simulink model "Zero"  (R2021b)
settings: Solver=VariableStepAuto  StartTime=0.0  StopTime=10.0  RelTol=1e-3
undefined symbols (not defined in the file): Newton, Raphson
libraries: simulink x12, slpidlib x1
settings Model: SimulationMode=accelerator  Creator=user  LastModifiedBy=cemery

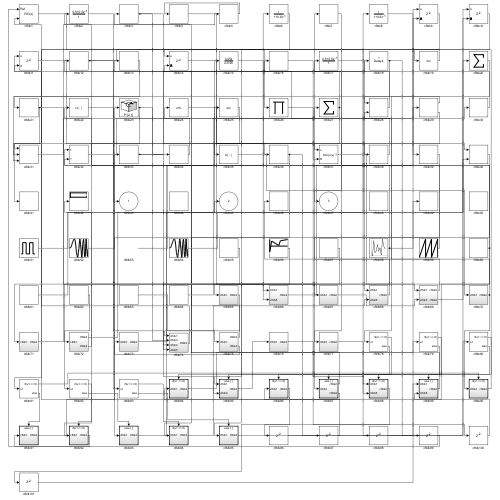
[thumbnail: Simulink's stored preview of the top-level diagram]
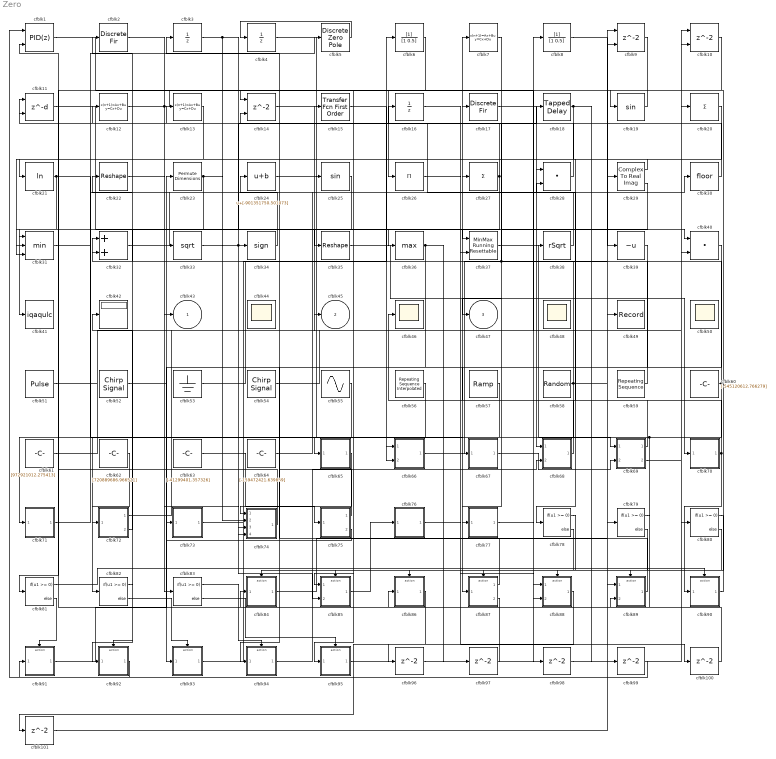
== system Zero ==
  cfblk1 : slpidlib/PID Controller (2DOF)  Controller=PID  Form=Parallel  TimeDomain=Discrete-time  UseExternalTs=off  SampleTime=1  IntegratorMethod=Forward Euler  FilterMethod=Forward Euler  ControllerParametersSource=internal  P=1  I=1  D=0  UseFilter=on  N=100  b=1  c=1  TunerSelectOption=Transfer Function Based (PID Tuner App)  InitialConditionSource=internal  InitialConditionForIntegrator=0  InitialConditionForFilter=0  DifferentiatorICPrevScaledInput=0  ExternalReset=none  TrackingMode=off  Kt=1  LimitOutput=off  SatLimitsSource=internal  UpperSaturationLimit=inf  LowerSaturationLimit=-inf  LinearizeAsGain=off  AntiWindupMode=none  Kb=1  POutMin=[]  POutMax=[]  IOutMin=[]  IOutMax=[]  DOutMin=[]  DOutMax=[]  NOutMin=[]  NOutMax=[]  bOutMin=[]  bOutMax=[]  cOutMin=[]  cOutMax=[]  SumOutMin=[]  SumOutMax=[]  SaturationOutMin=[]  SaturationOutMax=[]  PParamMin=[]  PParamMax=[]  IParamMin=[]  IParamMax=[]  DParamMin=[]  DParamMax=[]  NParamMin=[]  NParamMax=[]  bParamMin=[]  bParamMax=[]  cParamMin=[]  cParamMax=[]  KbParamMin=[]  KbParamMax=[]  KtParamMin=[]  KtParamMax=[]  KbOutMin=[]  KbOutMax=[]  KtOutMin=[]  KtOutMax=[]  IntegratorOutMin=[]  IntegratorOutMax=[]  FilterOutMin=[]  FilterOutMax=[]  SumI1OutMin=[]  SumI1OutMax=[]  SumI2OutMin=[]  SumI2OutMax=[]  SumI3OutMin=[]  SumI3OutMax=[]  SumI4OutMin=[]  SumI4OutMax=[]  SumDOutMin=[]  SumDOutMax=[]  Sum1OutMin=[]  Sum1OutMax=[]  Sum2OutMin=[]  Sum2OutMax=[]  Sum3OutMin=[]  Sum3OutMax=[]  DifferentiatorOutMin=[]  DifferentiatorOutMax=[]  FilterDiffOutCoefMin=[]  FilterDiffOutCoefMax=[]  ReciprocalOutMin=[]  ReciprocalOutMax=[]  SumDenOutMin=[]  SumDenOutMax=[]  SumNumOutMin=[]  SumNumOutMax=[]  DivideOutMin=[]  DivideOutMax=[]  UdiffTsProdOutMin=[]  UdiffTsProdOutMax=[]  NTsProdOutMin=[]  NTsProdOutMax=[]  UintegralTsProdOutMin=[]  UintegralTsProdOutMax=[]  UngainTsProdOutMin=[]  UngainTsProdOutMax=[]  IntegratorContinuousStateAttributes=''  IntegratorStateMustResolveToSignalObject=off  IntegratorRTWStateStorageClass=Auto  FilterContinuousStateAttributes=''  FilterStateMustResolveToSignalObject=off  FilterRTWStateStorageClass=Auto  ParallelPVariant=InternalParameters  IdealPVariant=Disabled  IVariant=InternalParameters  DVariant=InternalParameters  bVariant=InternalParameters  cVariant=InternalParameters  IntegratorVariant=Discrete  SatVariant=Disabled  AWVariant=Passthrough  PCopyVariant=Disabled  TRVariant=Disabled  FdbkBlocksVariant=Forward  IdealPFdbkVariant=Disabled  SatFdbkVariant=Disabled  DerivativeFilterVariant=ForwardEulerFilter  NVariant=InternalParameters  NCopyVariant=Disabled  FilterICVariant=InternalICsFilter  IntegratorICVariant=InternalICs  ExternalResetVariant=Disabled  TRSumVariant=Passthrough  SumFdbkVariant=Disabled  SumVariant=Sum_PID  TsampFilterVariant=InternalTs  TsampNgainVariant=Passthrough  TsampIntegralVariant=Passthrough  ExternalSaturationOutDataTypeStr=Inherit: Same as second input
      settings: SourceProductBaseCode=SL
  cfblk10 : Delay  ShowEnablePort=on  SampleTime=1
      settings: InputPortMap=u0,e6
  cfblk{96..101} (6 alike) : Delay  SampleTime=1
  cfblk11 : Delay  DelayLengthSource=Input port  SampleTime=1
      settings: InputPortMap=u0,p1
  cfblk12 : DiscreteStateSpace
  cfblk13 : DiscreteStateSpace
  cfblk14 : Delay  ShowEnablePort=on  SampleTime=1
      settings: InputPortMap=u0,e6
  cfblk15 : simulink/Discrete/Transfer Fcn First Order  PoleZ=0.95  ICPrevOutput=0.0  DoSatur=off
  cfblk16 : UnitDelay  HasFrameUpgradeWarning=on
  cfblk17 : DiscreteFir  SampleTime=1
  cfblk18 : simulink/Discrete/Tapped Delay  vinit=0.0  samptime=-1  NumDelays=1  DelayOrder=Oldest  includeCurrent=off
  cfblk19 : Trigonometry
  cfblk2 : DiscreteFir  SampleTime=1
  cfblk20 : Sum  Inputs=+
  cfblk21 : Math  Operator=log  SaturateOnIntegerOverflow=on
  cfblk22 : Reshape
  cfblk23 : PermuteDimensions
  cfblk24 : Bias  Bias=[-901351750.501073]
  cfblk25 : Trigonometry
  cfblk26 : Product  Inputs=*
  cfblk27 : Sum  Inputs=+
  cfblk28 : DotProduct  InputSameDT=on  OutDataTypeStr=Inherit: Inherit via internal rule
  cfblk29 : ComplexToRealImag
  cfblk3 : UnitDelay  HasFrameUpgradeWarning=on
  cfblk30 : Rounding
  cfblk31 : MinMax  Inputs=3
  cfblk32 : Sum
  cfblk33 : Sqrt  SaturateOnIntegerOverflow=on
  cfblk34 : Signum
  cfblk35 : Reshape
  cfblk36 : MinMax  Function=max
  cfblk37 : simulink/Math Operations/MinMax Running Resettable  Function=min  vinit=0.0
  cfblk38 : Sqrt  Operator=rSqrt  AlgorithmType=Newton-Raphson  SaturateOnIntegerOverflow=on
  cfblk39 : UnaryMinus
  cfblk4 : UnitDelay  HasFrameUpgradeWarning=on
  cfblk40 : DotProduct  InputSameDT=on  OutDataTypeStr=Inherit: Inherit via internal rule
  cfblk41 : ToWorkspace  VariableName=iqaqulc  SaveFormat=Timeseries  SampleTime=-1
  cfblk42 : Display
  cfblk{44,46,48,50} (4 alike) : Scope
      cfblk44 settings: Floating=on
      cfblk48 settings: Floating=on
      cfblk50 settings: Floating=on
  cfblk49 : Record  FileSettingsInternal="{\"entries\":[{\"content\":{\"excelSettings\":{\"content\":{},\"type\":\"Streamout.ExcelSettings\"}},\"type\":\"Streamout.FileSettingStorage\",\"uuid\":\"f2e1b8d2-99cf-47f0-99c0-b13258d1778a\"}],\"packageUris\":[\"http://schema.mathworks.com/mf0/streamout_blocks/R2020a\"],\"version\":\"1.0\"}"  SignalsInternal="{\"entries\":[{\"content\":{\"signals\":[{\"content\":{\"blockPath\":[\"sampleModel98/cfblk49\"],\"channel\":[],\"dimensions\":[1],\"domain\":\"sampleModel98/cfblk49\",\"lineColor\":\"#4dbeee\",\"plots\":[1],\"port\":1,\"sid\":[\"\"],\"signalID\":26449,\"signalName\":\"cfblk84\"},\"type\":\"RecordBlkView.Signal\",\"uuid\":\"a8dcc7f6-b363-4ce4-accc-3e93054832d9\"}]},\"type\":\"RecordBlkView.InputSignals\",\"uuid\":\"aaaac346-ddfa-4c10-a6ea-2fd00368ec74\"}],\"packageUris\":[\"http://schema.mathworks.com/mf0/streamout_blocks/R2020a\"],\"version\":\"1.0\"}"  VisualizationBindings="{\"sparklinesplugin\":{\"info\":[{\"bindingParametersList\":[],\"subplotID\":1}]}}"
  cfblk5 : DiscreteZeroPole  Poles=[0 0.5]  Gain=1
  cfblk51 : DiscretePulseGenerator  PulseType=Time based  Amplitude=[-833125303.274875]  Period=[62482245.083306]  PulseWidth=5  PhaseDelay=[3.000000]
  cfblk52 : simulink/Sources/Chirp Signal  f1=[698919112.611196]  T=[-838821150.471770]  f2=[519225321.163712]
  cfblk53 : Ground
  cfblk54 : simulink/Sources/Chirp Signal  f1=[387147427.874404]  T=[407726866.537460]  f2=[-675799982.541592]
  cfblk55 : Sin  Amplitude=[-344619677.755525]  Bias=[504210884.884345]  SampleTime=0
  cfblk56 : simulink/Sources/Repeating Sequence Interpolated  OutValues=[-768676903.120434, 734996835.272669, 105136173.110517, 743008723.110130, 950223410.347210]  TimeValues=[0 0.1 0.5 0.6 1].'  LookUpMeth=Use Input Below  tsamp=0.01  OutMin=[]  OutMax=[]  OutDataTypeStr=double  OutputDataTypeScalingMode=double  OutDataType=fixdt(0,8)  OutScaling=2^-10
  cfblk57 : simulink/Sources/Ramp  slope=[-4492.341158]  start=[1.599996]  InitialOutput=[910758.261460]
  cfblk58 : UniformRandomNumber  Minimum=[-3049811920.776981]  Maximum=[1513930273.771641]  Seed=[63448783.000000]  SampleTime=0.1
  cfblk59 : simulink/Sources/Repeating Sequence  rep_seq_t=[0 2]  rep_seq_y=[-591285366.145674, 872110472.793528]
  cfblk6 : DiscreteFilter  SampleTime=1
  cfblk60 : Constant  Value=[-545120612.766279]  SampleTime=1
  cfblk61 : Constant  Value=[972921012.275413]  SampleTime=1
  cfblk62 : Constant  Value=[720889686.966521]  SampleTime=1
  cfblk63 : Constant  Value=[-41299401.357326]  SampleTime=1
  cfblk64 : Constant  Value=[-159472421.639859]  SampleTime=1
  cfblk65 : Subsystem
  cfblk66 : Subsystem
  cfblk67 : Subsystem
  cfblk68 : Subsystem
  cfblk69 : Subsystem
  cfblk7 : DiscreteStateSpace
  cfblk70 : Subsystem
  cfblk71 : Subsystem
  cfblk72 : Subsystem
  cfblk73 : Subsystem
  cfblk74 : Subsystem
  cfblk75 : Subsystem
  cfblk76 : Subsystem
  cfblk77 : Subsystem
  cfblk{78..83} (6 alike) : If  IfExpression=u1 >= 0  SampleTime=1
  cfblk8 : DiscreteFilter  SampleTime=1
  cfblk84 : Subsystem  TreatAsAtomicUnit=on
  cfblk85 : Subsystem  TreatAsAtomicUnit=on
  cfblk86 : Subsystem  TreatAsAtomicUnit=on
  cfblk87 : Subsystem  TreatAsAtomicUnit=on
  cfblk88 : Subsystem  TreatAsAtomicUnit=on
  cfblk89 : Subsystem  TreatAsAtomicUnit=on
  cfblk9 : Delay  ShowEnablePort=on  SampleTime=1
      settings: InputPortMap=u0,e6
  cfblk90 : Subsystem  TreatAsAtomicUnit=on
  cfblk91 : Subsystem  TreatAsAtomicUnit=on
  cfblk92 : Subsystem  TreatAsAtomicUnit=on
  cfblk93 : Subsystem  TreatAsAtomicUnit=on
  cfblk94 : Subsystem  TreatAsAtomicUnit=on
  cfblk95 : Subsystem  TreatAsAtomicUnit=on
  cfblk43 : Outport
  cfblk45 : Outport  Port=2
  cfblk47 : Outport  Port=3
  wires:
  cfblk39/1 -> cfblk87/1(cfblk1)
  cfblk69/1(cfblk2) -> cfblk46/1
  cfblk62/1 -> cfblk82/1
  cfblk23/1 -> cfblk34/1, cfblk31/2
  cfblk68/1(cfblk2) -> cfblk7/1
  cfblk60/1 -> cfblk86/1(cfblk1), cfblk85/1(cfblk1), cfblk2/1, cfblk17/1
  cfblk14/1 -> cfblk40/1
  cfblk54/1 -> cfblk20/1
  cfblk12/1 -> cfblk26/1, cfblk74/4(cfblk5)
  cfblk35/1 -> cfblk70/1(cfblk1)
  cfblk5/1 -> cfblk4/1
  cfblk13/1 -> cfblk21/1
  cfblk17/1 -> cfblk68/1(cfblk1)
  cfblk20/1 -> cfblk78/1
  cfblk24/1 -> cfblk37/1
  cfblk85/1(cfblk2) -> cfblk76/1(cfblk1)
  cfblk34/1 -> cfblk24/1
  cfblk18/1 -> cfblk31/3, cfblk99/1
  cfblk63/1 -> cfblk75/1(cfblk1)
  cfblk33/1 -> cfblk18/1, cfblk85/2(cfblk4)
  cfblk90/1(cfblk2) -> cfblk19/1
  cfblk87/1(cfblk2) -> cfblk32/1
  cfblk66/1(cfblk2) -> cfblk9/1
  cfblk8/1 -> cfblk39/1
  cfblk4/1 -> cfblk67/1(cfblk1)
  cfblk56/1 -> cfblk72/1(cfblk1)
  cfblk6/1 -> cfblk95/1(cfblk1)
  cfblk3/1 -> cfblk36/1, cfblk74/2(cfblk3)
  cfblk40/1 -> cfblk93/1(cfblk1)
  cfblk61/1 -> cfblk8/1
  cfblk89/1(cfblk2) -> cfblk3/1
  cfblk52/1 -> cfblk23/1
  cfblk57/1 -> cfblk71/1(cfblk1)
  cfblk53/1 -> cfblk15/1
  cfblk11/1 -> cfblk66/1(cfblk1)
  cfblk38/1 -> cfblk16/1
  cfblk37/1 -> cfblk69/1(cfblk1)
  cfblk92/1(cfblk2) -> cfblk1/1
  cfblk32/1 -> cfblk9/2
  cfblk73/1(cfblk2) -> cfblk6/1
  cfblk70/1(cfblk2) -> cfblk90/1(cfblk1), cfblk28/2
  cfblk15/1 -> cfblk38/1
  cfblk51/1 -> cfblk10/1
  cfblk91/1(cfblk2) -> cfblk33/1
  cfblk22/1 -> cfblk43/1
  cfblk21/1 -> cfblk41/1, cfblk66/2(cfblk5)
  cfblk28/1 -> cfblk13/1
  cfblk55/1 -> cfblk65/1(cfblk1)
  cfblk71/1(cfblk2) -> cfblk27/1
  cfblk74/1(cfblk2) -> cfblk11/1
  cfblk36/1 -> cfblk94/1(cfblk1), cfblk97/1
  cfblk72/1(cfblk2) -> cfblk25/1
  cfblk2/1 -> cfblk83/1
  cfblk67/1(cfblk2) -> cfblk69/2(cfblk3)
  cfblk31/1 -> cfblk5/1
  cfblk30/1 -> cfblk12/1
  cfblk1/1 -> cfblk88/1(cfblk1)
  cfblk26/1 -> cfblk88/2(cfblk5)
  cfblk9/1 -> cfblk81/1
  cfblk29/1 -> cfblk28/1
  cfblk16/1 -> cfblk37/2
  cfblk93/1(cfblk2) -> cfblk45/1
  cfblk94/1(cfblk2) -> cfblk68/2(cfblk5)
  cfblk25/1 -> cfblk35/1
  cfblk10/1 -> cfblk31/1
  cfblk19/1 -> cfblk14/1
  cfblk59/1 -> cfblk32/2
  cfblk65/1(cfblk2) -> cfblk74/1(cfblk1)
  cfblk29/2 -> cfblk47/1
  cfblk64/1 -> cfblk30/1
  cfblk95/1(cfblk2) -> cfblk10/2
  cfblk7/1 -> cfblk77/1(cfblk1)
  cfblk58/1 -> cfblk29/1, cfblk22/1, cfblk74/3(cfblk4)
  cfblk72/2(cfblk4) -> cfblk42/1
  cfblk27/1 -> cfblk92/1(cfblk1), cfblk11/2
  cfblk87/2(cfblk4) -> cfblk84/1(cfblk1)
  cfblk69/2(cfblk4) -> cfblk40/2
  cfblk84/1(cfblk2) -> cfblk49/1
  cfblk75/1(cfblk2) -> cfblk14/2
  cfblk75/2(cfblk4) -> cfblk73/1(cfblk1)
  cfblk78/1 -> cfblk84/Action
  cfblk78/2 -> cfblk85/Action
  cfblk79/1 -> cfblk86/Action
  cfblk79/2 -> cfblk87/Action
  cfblk80/1 -> cfblk88/Action
  cfblk80/2 -> cfblk89/Action
  cfblk81/1 -> cfblk90/Action
  cfblk81/2 -> cfblk91/Action
  cfblk82/1 -> cfblk92/Action
  cfblk82/2 -> cfblk93/Action
  cfblk83/1 -> cfblk94/Action
  cfblk83/2 -> cfblk95/Action
  cfblk88/1(cfblk2) -> cfblk96/1
  cfblk96/1 -> cfblk80/1
  cfblk97/1 -> cfblk1/2
  cfblk77/1(cfblk2) -> cfblk98/1
  cfblk98/1 -> cfblk89/1(cfblk1)
  cfblk99/1 -> cfblk91/1(cfblk1)
  cfblk76/1(cfblk2) -> cfblk100/1
  cfblk100/1 -> cfblk89/2(cfblk5)
  cfblk86/1(cfblk2) -> cfblk101/1
  cfblk101/1 -> cfblk79/1

== system Zero/cfblk65 ==
  cfblk1 : Inport
  cfblk3 : UnaryMinus
  cfblk2 : Outport
  wires:
  cfblk1/1 -> cfblk2/1, cfblk3/1

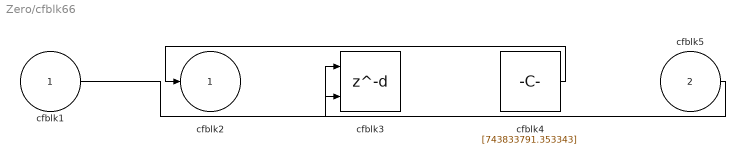
== system Zero/cfblk66 ==
  cfblk1 : Inport
  cfblk5 : Inport  Port=2
  cfblk3 : Delay  DelayLengthSource=Input port  SampleTime=1
      settings: InputPortMap=u0,p1
  cfblk4 : Constant  Value=[743833791.353343]  SampleTime=1
  cfblk2 : Outport
  wires:
  cfblk4/1 -> cfblk2/1
  cfblk5/1 -> cfblk3/1
  cfblk1/1 -> cfblk3/2

== system Zero/cfblk67 ==
  cfblk1 : Inport
  cfblk3 : Polyval  Coefs=[ +2.081618890e-019, -1.441693666e-014, +4.719686976e-010, -8.536869453e-006, +1.621573104e-001, -8.087801117e+001 ]
  cfblk2 : Outport
  wires:
  cfblk1/1 -> cfblk3/1
  cfblk3/1 -> cfblk2/1

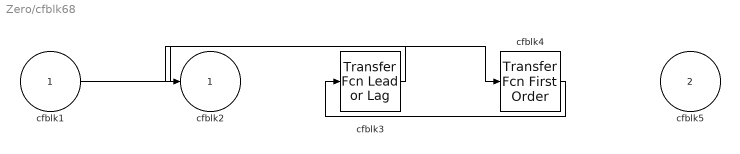
== system Zero/cfblk68 ==
  cfblk1 : Inport
  cfblk5 : Inport  Port=2
  cfblk3 : simulink/Discrete/Transfer Fcn Lead or Lag  PoleZ=0.95  ZeroZ=0.75  ICPrevOutput=0.0  ICPrevInput=0.0  DoSatur=off
      settings: SourceProductBaseCode=SL
  cfblk4 : simulink/Discrete/Transfer Fcn First Order  PoleZ=0.95  ICPrevOutput=0.0  DoSatur=off
  cfblk2 : Outport
  wires:
  cfblk1/1 -> cfblk4/1
  cfblk4/1 -> cfblk3/1
  cfblk3/1 -> cfblk2/1

== system Zero/cfblk69 ==
  cfblk1 : Inport
  cfblk3 : Inport  Port=2
  cfblk2 : Outport
  cfblk4 : Outport  Port=2
  wires:
  cfblk3/1 -> cfblk4/1
  cfblk1/1 -> cfblk2/1

== system Zero/cfblk70 ==
  cfblk1 : Inport
  cfblk3 : simulink/Discrete/Transfer Fcn Real Zero  ZeroZ=0.75  ICPrevInput=0.0  DoSatur=off
      settings: SourceProductBaseCode=SL
  cfblk2 : Outport
  wires:
  cfblk1/1 -> cfblk2/1, cfblk3/1

== system Zero/cfblk71 ==
  cfblk1 : Inport
  cfblk3 : simulink/Discrete/Tapped Delay  vinit=0.0  samptime=-1  NumDelays=1  DelayOrder=Oldest  includeCurrent=off
  cfblk4 : Constant  Value=[-493454779.766346]  SampleTime=1
  cfblk2 : Outport
  wires:
  cfblk4/1 -> cfblk2/1
  cfblk1/1 -> cfblk3/1

== system Zero/cfblk72 ==
  cfblk1 : Inport
  cfblk3 : Sum  Inputs=-+
  cfblk2 : Outport
  cfblk4 : Outport  Port=2
  wires:
  cfblk3/1 -> cfblk2/1
  cfblk1/1 -> cfblk4/1, cfblk3/1, cfblk3/2

== system Zero/cfblk73 ==
  cfblk1 : Inport
  cfblk3 : DiscreteFir  SampleTime=1
  cfblk4 : Squeeze
  cfblk2 : Outport
  wires:
  cfblk1/1 -> cfblk4/1
  cfblk4/1 -> cfblk3/1
  cfblk3/1 -> cfblk2/1

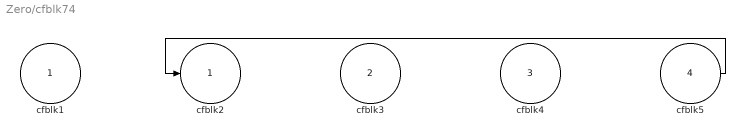
== system Zero/cfblk74 ==
  cfblk1 : Inport
  cfblk3 : Inport  Port=2
  cfblk4 : Inport  Port=3
  cfblk5 : Inport  Port=4
  cfblk2 : Outport
  wires:
  cfblk5/1 -> cfblk2/1

== system Zero/cfblk75 ==
  cfblk1 : Inport
  cfblk3 : Gain  Gain=[733775026.477658]
  cfblk2 : Outport
  cfblk4 : Outport  Port=2
  wires:
  cfblk1/1 -> cfblk2/1, cfblk3/1
  cfblk3/1 -> cfblk4/1

== system Zero/cfblk76 ==
  cfblk1 : Inport
  cfblk3 : Gain  Gain=[842656306.747362]
  cfblk2 : Outport
  wires:
  cfblk1/1 -> cfblk3/1
  cfblk3/1 -> cfblk2/1

== system Zero/cfblk77 ==
  cfblk1 : Inport
  cfblk3 : Sum  Inputs=+-
  cfblk2 : Outport
  wires:
  cfblk1/1 -> cfblk2/1, cfblk3/1, cfblk3/2

== system Zero/cfblk84 ==
  cfblk1 : Inport
  Action Port : ActionPort  ActionPortLabel=if(u1 >= 0)
  cfblk3 : Reshape
  cfblk2 : Outport
  wires:
  cfblk1/1 -> cfblk2/1, cfblk3/1

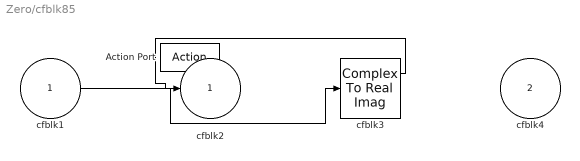
== system Zero/cfblk85 ==
  cfblk1 : Inport
  cfblk4 : Inport  Port=2
  Action Port : ActionPort  ActionPortLabel=else
  cfblk3 : ComplexToRealImag
  cfblk2 : Outport
  wires:
  cfblk1/1 -> cfblk3/1
  cfblk3/1 -> cfblk2/1

== system Zero/cfblk86 ==
  cfblk1 : Inport
  Action Port : ActionPort  ActionPortLabel=if(u1 >= 0)
  cfblk3 : MinMax
  cfblk2 : Outport
  wires:
  cfblk3/1 -> cfblk2/1
  cfblk1/1 -> cfblk3/1

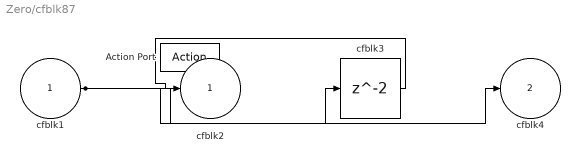
== system Zero/cfblk87 ==
  cfblk1 : Inport
  Action Port : ActionPort  ActionPortLabel=else
  cfblk3 : Delay
  cfblk2 : Outport
  cfblk4 : Outport  Port=2
  wires:
  cfblk1/1 -> cfblk4/1, cfblk3/1
  cfblk3/1 -> cfblk2/1

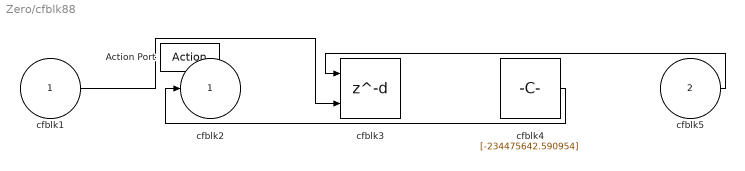
== system Zero/cfblk88 ==
  cfblk1 : Inport
  cfblk5 : Inport  Port=2
  Action Port : ActionPort  ActionPortLabel=if(u1 >= 0)
  cfblk3 : Delay  DelayLengthSource=Input port
      settings: InputPortMap=u0,p1
  cfblk4 : Constant  Value=[-234475642.590954]  SampleTime=1
  cfblk2 : Outport
  wires:
  cfblk4/1 -> cfblk2/1
  cfblk5/1 -> cfblk3/1
  cfblk1/1 -> cfblk3/2

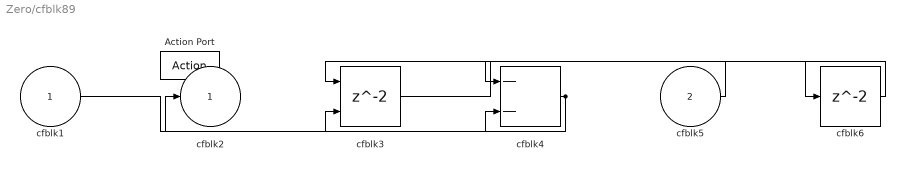
== system Zero/cfblk89 ==
  cfblk1 : Inport
  cfblk5 : Inport  Port=2
  Action Port : ActionPort  ActionPortLabel=else
  cfblk3 : Delay  ShowEnablePort=on
      settings: InputPortMap=u0,e6
  cfblk4 : Sum  Inputs=--
  cfblk6 : Delay
  cfblk2 : Outport
  wires:
  cfblk4/1 -> cfblk2/1, cfblk3/2
  cfblk1/1 -> cfblk4/2
  cfblk5/1 -> cfblk3/1
  cfblk3/1 -> cfblk6/1
  cfblk6/1 -> cfblk4/1

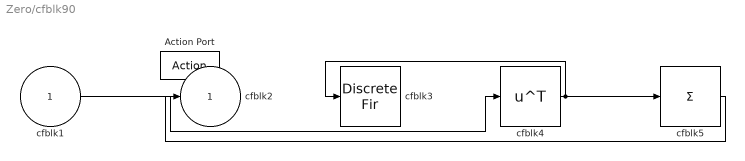
== system Zero/cfblk90 ==
  cfblk1 : Inport
  Action Port : ActionPort  ActionPortLabel=if(u1 >= 0)
  cfblk3 : DiscreteFir
  cfblk4 : Math  Operator=transpose  SaturateOnIntegerOverflow=on
  cfblk5 : Sum  Inputs=+
  cfblk2 : Outport
  wires:
  cfblk1/1 -> cfblk4/1
  cfblk5/1 -> cfblk2/1
  cfblk4/1 -> cfblk5/1, cfblk3/1

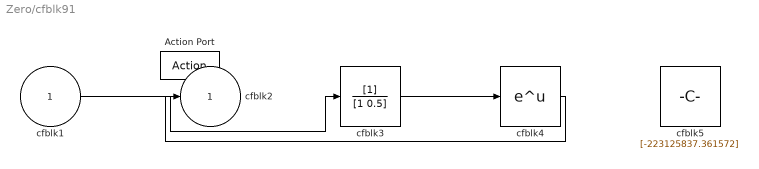
== system Zero/cfblk91 ==
  cfblk1 : Inport
  Action Port : ActionPort  ActionPortLabel=else
  cfblk3 : DiscreteFilter
  cfblk4 : Math  SaturateOnIntegerOverflow=on
  cfblk5 : Constant  Value=[-223125837.361572]  SampleTime=1
  cfblk2 : Outport
  wires:
  cfblk1/1 -> cfblk3/1
  cfblk3/1 -> cfblk4/1
  cfblk4/1 -> cfblk2/1

== system Zero/cfblk92 ==
  cfblk1 : Inport
  Action Port : ActionPort  ActionPortLabel=if(u1 >= 0)
  cfblk3 : DiscreteFir
  cfblk2 : Outport
  wires:
  cfblk3/1 -> cfblk2/1
  cfblk1/1 -> cfblk3/1

== system Zero/cfblk93 ==
  cfblk1 : Inport
  Action Port : ActionPort  ActionPortLabel=else
  cfblk3 : Sqrt  Operator=rSqrt  AlgorithmType=Newton-Raphson  SaturateOnIntegerOverflow=on
  cfblk2 : Outport
  wires:
  cfblk3/1 -> cfblk2/1
  cfblk1/1 -> cfblk3/1

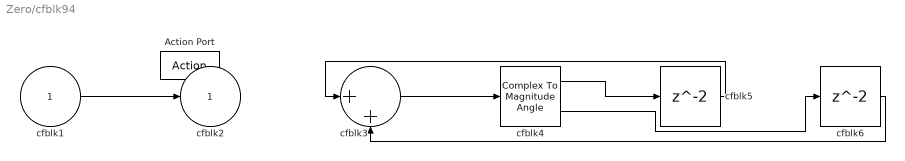
== system Zero/cfblk94 ==
  cfblk1 : Inport
  Action Port : ActionPort  ActionPortLabel=if(u1 >= 0)
  cfblk3 : Sum  Inputs=|++
  cfblk4 : ComplexToMagnitudeAngle
  cfblk5 : Delay
  cfblk6 : Delay
  cfblk2 : Outport
  wires:
  cfblk3/1 -> cfblk4/1
  cfblk1/1 -> cfblk2/1
  cfblk4/1 -> cfblk5/1
  cfblk5/1 -> cfblk3/1
  cfblk4/2 -> cfblk6/1
  cfblk6/1 -> cfblk3/2

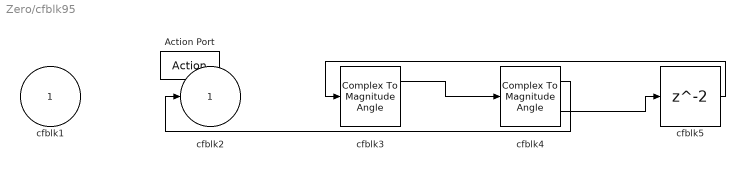
== system Zero/cfblk95 ==
  cfblk1 : Inport
  Action Port : ActionPort  ActionPortLabel=else
  cfblk3 : ComplexToMagnitudeAngle
  cfblk4 : ComplexToMagnitudeAngle
  cfblk5 : Delay
  cfblk2 : Outport
  wires:
  cfblk3/1 -> cfblk4/1
  cfblk4/1 -> cfblk2/1
  cfblk4/2 -> cfblk5/1
  cfblk5/1 -> cfblk3/1
